simulink model "cubesat_attitude_3axis"  (R2025b)
settings: Solver=ode45  StartTime=0.0  StopTime=simulation_duration_3axis  RelTol=1e-8  AbsTol=1e-10
values from neighbouring files (symbols this model uses):
  command_quaternion_3axis = euler_to_quaternion(commanded_attitude_3axis)    [init_simulink_3axis.m]
  I = diag([Ixx, Iyy, Izz])    [init_attitude_3axis.m]    (also in init_attitude_3axis_asymmetric.m)
  initial_state_3axis = [ ... (first row only)    [init_simulink_3axis.m]
  Kd_3axis = reference_Kd      * principal_inertia / reference_inertia    [init_simulink_3axis.m]
  Kp_3axis = reference_Kp      * principal_inertia / reference_inertia    [init_simulink_3axis.m]
  wheel_inertia = [ ... (first row only)    [init_reaction_wheels.m]    (also in magnetorquer_momentum_dump.m = wheel_inertia(:))
  wheel_speed_max = wheel_speed_max_rpm * 2*pi / 60    [init_reaction_wheels.m]
  wheel_torque_max = [ ... (first row only)    [init_reaction_wheels.m]
settings Model: Creator=matho  LastModifiedBy=matho

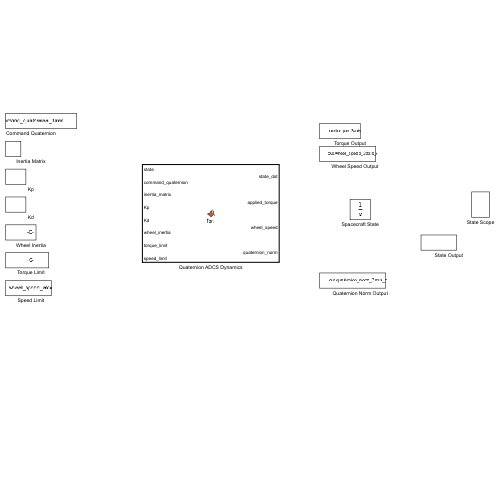
[thumbnail: Simulink's stored preview of the top-level diagram]
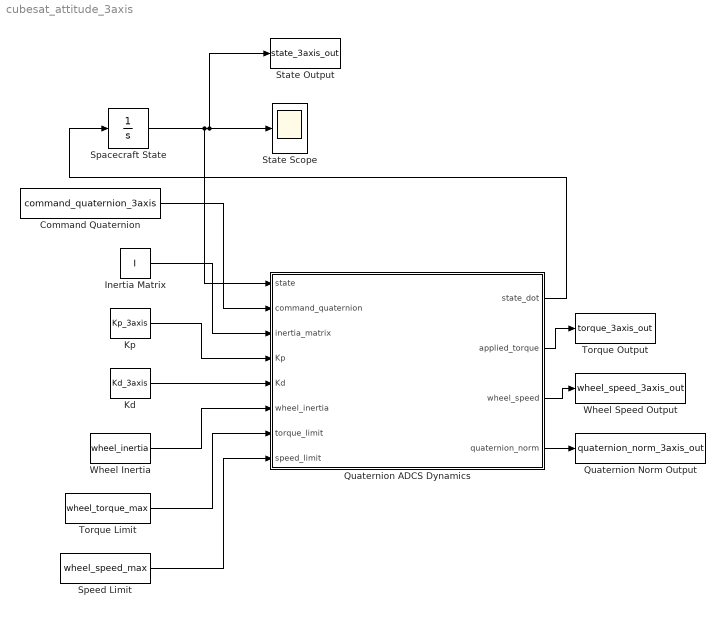
== system cubesat_attitude_3axis ==
  Command Quaternion : Constant  Value=command_quaternion_3axis
  Inertia Matrix : Constant  Value=I
  Kd : Constant  Value=Kd_3axis
  Kp : Constant  Value=Kp_3axis
  Quaternion ADCS Dynamics : MATLAB Function  TreatAsAtomicUnit=on
  Quaternion Norm Output : ToWorkspace  VariableName=quaternion_norm_3axis_out  SaveFormat=Timeseries  SampleTime=-1
  Spacecraft State : Integrator  InitialCondition=initial_state_3axis
  Speed Limit : Constant  Value=wheel_speed_max
  State Output : ToWorkspace  VariableName=state_3axis_out  SaveFormat=Timeseries  SampleTime=-1
  State Scope : Scope
  Torque Limit : Constant  Value=wheel_torque_max
  Torque Output : ToWorkspace  VariableName=torque_3axis_out  SaveFormat=Timeseries  SampleTime=-1
  Wheel Inertia : Constant  Value=wheel_inertia
  Wheel Speed Output : ToWorkspace  VariableName=wheel_speed_3axis_out  SaveFormat=Timeseries  SampleTime=-1
  wires:
  Spacecraft State/1 -> State Output/1, State Scope/1, Quaternion ADCS Dynamics/1(state)
  Command Quaternion/1 -> Quaternion ADCS Dynamics/2(command_quaternion)
  Kp/1 -> Quaternion ADCS Dynamics/4(Kp)
  Inertia Matrix/1 -> Quaternion ADCS Dynamics/3(inertia_matrix)
  Wheel Inertia/1 -> Quaternion ADCS Dynamics/6(wheel_inertia)
  Speed Limit/1 -> Quaternion ADCS Dynamics/8(speed_limit)
  Kd/1 -> Quaternion ADCS Dynamics/5(Kd)
  Torque Limit/1 -> Quaternion ADCS Dynamics/7(torque_limit)
  Quaternion ADCS Dynamics/1(state_dot) -> Spacecraft State/1
  Quaternion ADCS Dynamics/2(applied_torque) -> Torque Output/1
  Quaternion ADCS Dynamics/3(wheel_speed) -> Wheel Speed Output/1
  Quaternion ADCS Dynamics/4(quaternion_norm) -> Quaternion Norm Output/1

== matlab function cubesat_attitude_3axis/Quaternion ADCS Dynamics ==
  data: state input; state_dot output; command_quaternion input; inertia_matrix input; Kp input; Kd input; wheel_inertia input; torque_limit input; speed_limit input; applied_torque output; wheel_speed output; quaternion_norm output
function [state_dot, applied_torque, wheel_speed, quaternion_norm] = fcn(state, command_quaternion, inertia_matrix, Kp, Kd, wheel_inertia, torque_limit, speed_limit)
%#codegen

quaternion = state(1:4);
body_rate = state(5:7);
wheel_speed = state(8:10);

[~, requested_torque] = pd_controller_quaternion( ...
    command_quaternion, quaternion, body_rate, ...
    Kp, Kd, torque_limit);

[applied_torque, wheel_acceleration] = ...
    reaction_wheel_actuator( ...
        requested_torque, wheel_speed, ...
        wheel_inertia, torque_limit, speed_limit);

quaternion_dot = quaternion_kinematics( ...
    quaternion, body_rate);

total_body_momentum = ...
    inertia_matrix * body_rate ...
    + wheel_inertia .* wheel_speed;

body_rate_dot = inertia_matrix \ ( ...
    applied_torque ...
    - cross(body_rate, total_body_momentum));

state_dot = [ ...
    quaternion_dot; ...
    body_rate_dot; ...
    wheel_acceleration];

quaternion_norm = sqrt(sum(quaternion.^2));
end
